simulink model "comparando_simulacoes_rate_diferente_entre_sensor_e_controlador"  (R2012b)
settings: Solver=ode3  StartTime=0.0  StopTime=1  FixedStep=1e-5  RelTol=1e-6
undefined symbols (not defined in the file): J, Kd, Ke, Kt, L, P, R
libraries: simulink x86
(part 2 of 3)

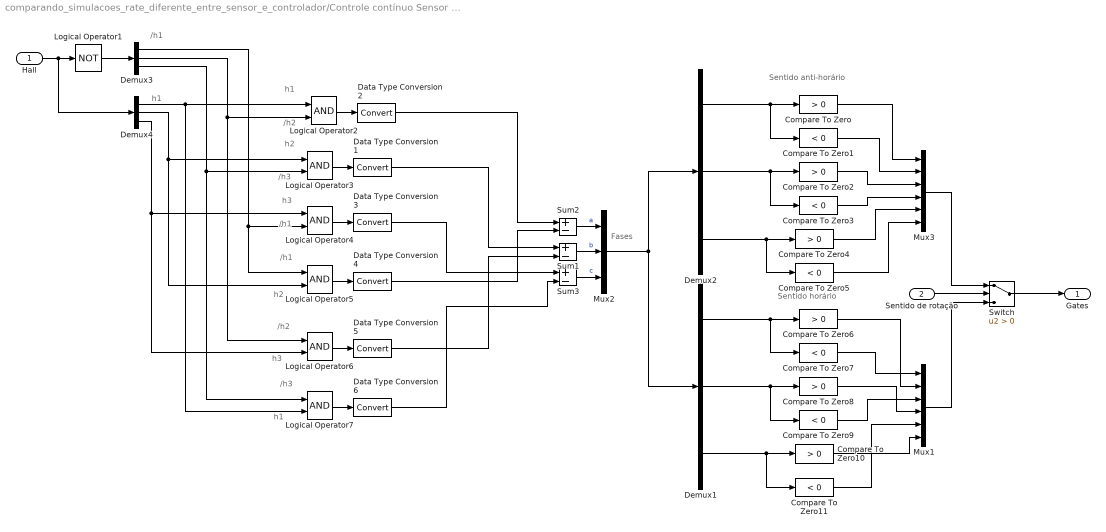
== system comparando_simulacoes_rate_diferente_entre_sensor_e_controlador/Controle contínuo Sensor instantâneo/Decoder ==
  note: Fases
  note: Sentido horário
  note: Sentido anti-horário
  note: h1
  note: /h3
  note: h3
  note: /h2
  note: h2
  note: /h1
  note: /h1
  note: h3
  note: /h3
  note: h2
  note: /h2
  note: h1
  note: h1
  note: /h1
  "Hall " : Inport
  Sentido de rotação : Inport  Port=2
  Compare To Zero{,2,4,6,8,10} (6 alike) : simulink/Logic and Bit Operations/Compare To Zero  relop=>  OutDataTypeStr=boolean  ZeroCross=off
  Compare To Zero{1,3,5,7,9,11} (6 alike) : simulink/Logic and Bit Operations/Compare To Zero  relop=<  OutDataTypeStr=boolean  ZeroCross=off
  Data Type Conversion{1..6} (6 alike) : DataTypeConversion
  Demux{1..4} (4 alike) : Demux  Outputs=3
  Logical Operator1 : Logic  Operator=NOT  AllPortsSameDT=off  OutDataTypeStr=boolean
  Logical Operator{2..7} (6 alike) : Logic  AllPortsSameDT=off  OutDataTypeStr=boolean
  Mux1 : Mux  Inputs=6
  Mux2 : Mux  Inputs=3
  Mux3 : Mux  Inputs=6
  Sum1 : Sum  Inputs=+-  OutDataTypeStr=double
  Sum2 : Sum  Inputs=+-  OutDataTypeStr=double
  Sum3 : Sum  Inputs=+-  OutDataTypeStr=double
  Switch : Switch  Criteria=u2 > Threshold
  Gates : Outport
  wires:
  Mux2/1 -> Demux1/1, Demux2/1
  Data Type Conversion6/1 -> Sum3/2
  Data Type Conversion3/1 -> Sum3/1
  Data Type Conversion5/1 -> Sum1/2
  Data Type Conversion1/1 -> Sum1/1
  Data Type Conversion4/1 -> Sum2/2
  Data Type Conversion2/1 -> Sum2/1
  Logical Operator7/1 -> Data Type Conversion6/1
  Logical Operator6/1 -> Data Type Conversion5/1
  Logical Operator5/1 -> Data Type Conversion4/1
  Logical Operator4/1 -> Data Type Conversion3/1
  Logical Operator3/1 -> Data Type Conversion1/1
  Sum3/1 -> Mux2/3  "c"
  Sum1/1 -> Mux2/2  "b"
  Sum2/1 -> Mux2/1  "a"
  Logical Operator2/1 -> Data Type Conversion2/1
  Demux3/1 -> Logical Operator5/1, Logical Operator4/2
  Demux3/2 -> Logical Operator6/1, Logical Operator2/2
  Demux3/3 -> Logical Operator7/1, Logical Operator3/2
  Demux4/1 -> Logical Operator7/2, Logical Operator2/1
  Demux4/2 -> Logical Operator5/2, Logical Operator3/1
  Demux4/3 -> Logical Operator6/2, Logical Operator4/1
  Logical Operator1/1 -> Demux3/1
  "Hall "/1 -> Demux4/1, Logical Operator1/1
  Compare To Zero10/1 -> Mux1/6
  Compare To Zero11/1 -> Mux1/5
  Compare To Zero8/1 -> Mux1/4
  Compare To Zero9/1 -> Mux1/3
  Compare To Zero6/1 -> Mux1/2
  Compare To Zero7/1 -> Mux1/1
  Switch/1 -> Gates/1
  Mux1/1 -> Switch/3
  Sentido de rotação/1 -> Switch/2
  Mux3/1 -> Switch/1
  Demux1/3 -> Compare To Zero11/1, Compare To Zero10/1
  Demux1/2 -> Compare To Zero9/1, Compare To Zero8/1
  Demux1/1 -> Compare To Zero7/1, Compare To Zero6/1
  Compare To Zero5/1 -> Mux3/6
  Compare To Zero4/1 -> Mux3/5
  Compare To Zero3/1 -> Mux3/4
  Compare To Zero2/1 -> Mux3/3
  Compare To Zero1/1 -> Mux3/2
  Compare To Zero/1 -> Mux3/1
  Demux2/3 -> Compare To Zero5/1, Compare To Zero4/1
  Demux2/2 -> Compare To Zero3/1, Compare To Zero2/1
  Demux2/1 -> Compare To Zero1/1, Compare To Zero/1

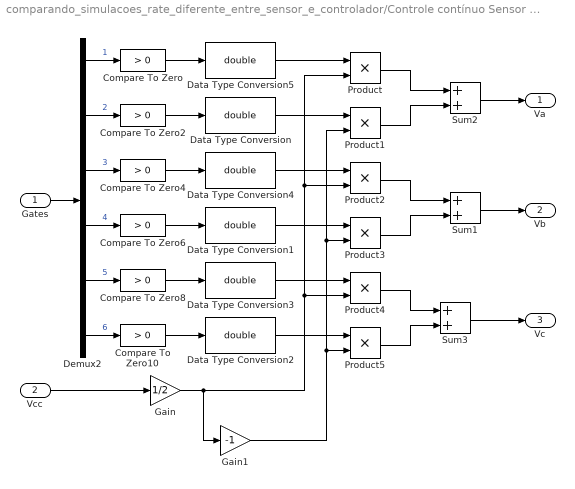
== system comparando_simulacoes_rate_diferente_entre_sensor_e_controlador/Controle contínuo Sensor instantâneo/Inversor ==
  Gates : Inport
  Vcc : Inport  Port=2
  Compare To Zero : simulink/Logic and Bit Operations/Compare To Zero  relop=>  OutDataTypeStr=uint8  ZeroCross=off
  Compare To Zero{2,6,8,10} (4 alike) : simulink/Logic and Bit Operations/Compare To Zero  relop=>  OutDataTypeStr=boolean  ZeroCross=off
  Compare To Zero4 : simulink/Logic and Bit Operations/Compare To Zero  relop=>  OutDataTypeStr=uint8  ZeroCross=off
  Data Type Conversion{,1..5} (6 alike) : DataTypeConversion  OutDataTypeStr=double
  Demux2 : Demux  Outputs=6
  Gain : Gain  Gain=1/2
  Gain1 : Gain  Gain=-1
  Product{,1..5} (6 alike) : Product  RndMeth=Zero
  Sum1 : Sum  SaturateOnIntegerOverflow=on
  Sum2 : Sum  SaturateOnIntegerOverflow=on
  Sum3 : Sum  SaturateOnIntegerOverflow=on
  Va : Outport
  Vb : Outport  Port=2
  Vc : Outport  Port=3
  wires:
  Vcc/1 -> Gain/1
  Sum1/1 -> Vb/1
  Sum3/1 -> Vc/1
  Sum2/1 -> Va/1
  Gates/1 -> Demux2/1
  Demux2/1 -> Compare To Zero/1  "1"
  Demux2/2 -> Compare To Zero2/1  "2"
  Demux2/3 -> Compare To Zero4/1  "3"
  Demux2/4 -> Compare To Zero6/1  "4"
  Demux2/5 -> Compare To Zero8/1  "5"
  Demux2/6 -> Compare To Zero10/1  "6"
  Compare To Zero/1 -> Data Type Conversion5/1
  Compare To Zero2/1 -> Data Type Conversion/1
  Compare To Zero4/1 -> Data Type Conversion4/1
  Compare To Zero6/1 -> Data Type Conversion1/1
  Compare To Zero8/1 -> Data Type Conversion3/1
  Compare To Zero10/1 -> Data Type Conversion2/1
  Product/1 -> Sum2/1
  Product1/1 -> Sum2/2
  Product2/1 -> Sum1/1
  Product3/1 -> Sum1/2
  Product4/1 -> Sum3/1
  Product5/1 -> Sum3/2
  Data Type Conversion2/1 -> Product5/1
  Data Type Conversion3/1 -> Product4/1
  Data Type Conversion1/1 -> Product3/1
  Data Type Conversion4/1 -> Product2/1
  Data Type Conversion/1 -> Product1/1
  Data Type Conversion5/1 -> Product/1
  Gain1/1 -> Product5/2, Product3/2, Product1/2
  Gain/1 -> Gain1/1, Product4/2, Product2/2, Product/2

== system comparando_simulacoes_rate_diferente_entre_sensor_e_controlador/Controle contínuo Sensor instantâneo/Sensores Hall ==
  teta_e : Inport
  Constant10 : Constant  Value=240
  Constant11 : Constant  Value=360
  Constant12 : Constant  Value=180
  Constant6 : Constant  Value=0
  Constant7 : Constant  Value=120
  Constant8 : Constant  Value=300
  Constant9 : Constant  Value=60
  Data Type Conversion3 : DataTypeConversion  SaturateOnIntegerOverflow=on  RndMeth=Zero
  Data Type Conversion4 : DataTypeConversion  SaturateOnIntegerOverflow=on  RndMeth=Zero
  Data Type Conversion5 : DataTypeConversion  SaturateOnIntegerOverflow=on  RndMeth=Zero
  Gain1 : Gain  Gain=180/pi
  Logical Operator3 : Logic  AllPortsSameDT=off  OutDataTypeStr=boolean
  Logical Operator4 : Logic  Operator=OR  AllPortsSameDT=off  OutDataTypeStr=boolean
  Logical Operator5 : Logic  AllPortsSameDT=off  OutDataTypeStr=boolean
  Math Function1 : Math  Operator=mod  SaturateOnIntegerOverflow=on
  Mux1 : Mux  Inputs=3
  Relational Operator{7,9..10,12} (4 alike) : RelationalOperator  InputSameDT=on
  Relational Operator11 : RelationalOperator  Operator=<=  InputSameDT=on
  Relational Operator8 : RelationalOperator  Operator=<=  InputSameDT=on
  Hall : Outport
  wires:
  teta_e/1 -> Gain1/1
  Constant6/1 -> Relational Operator7/2
  Constant7/1 -> Relational Operator8/2
  Constant8/1 -> Relational Operator9/2
  Relational Operator9/1 -> Logical Operator4/2
  Logical Operator3/1 -> Logical Operator4/1
  Relational Operator7/1 -> Logical Operator3/1
  Relational Operator8/1 -> Logical Operator3/2
  Relational Operator10/1 -> Logical Operator5/1
  Relational Operator11/1 -> Logical Operator5/2
  Constant9/1 -> Relational Operator10/2
  Constant10/1 -> Relational Operator11/2
  Constant12/1 -> Relational Operator12/2
  Mux1/1 -> Hall/1
  Data Type Conversion3/1 -> Mux1/1
  Data Type Conversion4/1 -> Mux1/2
  Data Type Conversion5/1 -> Mux1/3
  Logical Operator4/1 -> Data Type Conversion3/1
  Logical Operator5/1 -> Data Type Conversion4/1
  Relational Operator12/1 -> Data Type Conversion5/1
  Gain1/1 -> Math Function1/1
  Constant11/1 -> Math Function1/2
  Math Function1/1 -> Relational Operator8/1, Relational Operator9/1, Relational Operator10/1, Relational Operator11/1, Relational Operator12/1, Relational Operator7/1

== system comparando_simulacoes_rate_diferente_entre_sensor_e_controlador/Controlador contínuo Sensor discreto M (Ts = 0.01)/BLDC1/Cálculo Torque fase "a" ==
  i_a : Inport
  Theta_e : Inport  Port=2
  Constant1 : Constant  Value=360
  Gain : Gain  Gain=Kt/2
  Gain1 : Gain  Gain=180/pi
  Math Function1 : Math  Operator=mod  SaturateOnIntegerOverflow=on
  Product : Product  RndMeth=Zero
  fa1 : Lookup  InputValues=[0 30 60 90 120 150 180 210 240 270 300 330 360]  Table=[ 1 1 1 0 -1 -1 -1 -1 -1 0 1 1 1]
  T_a : Outport
  wires:
  i_a/1 -> Gain/1
  Gain/1 -> Product/2
  Math Function1/1 -> fa1/1
  Theta_e/1 -> Gain1/1
  fa1/1 -> Product/1
  Product/1 -> T_a/1
  Gain1/1 -> Math Function1/1
  Constant1/1 -> Math Function1/2

== system comparando_simulacoes_rate_diferente_entre_sensor_e_controlador/Controlador contínuo Sensor discreto M (Ts = 0.01)/BLDC1/Cálculo Torque fase "b" ==
  i_b : Inport
  Theta_e : Inport  Port=2
  Constant1 : Constant  Value=360
  Gain : Gain  Gain=Kt/2
  Gain1 : Gain  Gain=180/pi
  Math Function1 : Math  Operator=mod  SaturateOnIntegerOverflow=on
  Product : Product  RndMeth=Zero
  fb2 : Lookup  InputValues=[0 30 60 90 120 150 180 210 240 270 300 330 360]  Table=[-1 0 1 1 1 1 1 0 -1 -1 -1 -1 -1]
  T_b : Outport
  wires:
  Product/1 -> T_b/1
  fb2/1 -> Product/1
  Theta_e/1 -> Gain1/1
  Math Function1/1 -> fb2/1
  Gain/1 -> Product/2
  i_b/1 -> Gain/1
  Gain1/1 -> Math Function1/1
  Constant1/1 -> Math Function1/2

== system comparando_simulacoes_rate_diferente_entre_sensor_e_controlador/Controlador contínuo Sensor discreto M (Ts = 0.01)/BLDC1/Cálculo Torque fase "c" ==
  i_c : Inport
  Theta_e : Inport  Port=2
  Constant1 : Constant  Value=360
  Gain : Gain  Gain=Kt/2
  Gain1 : Gain  Gain=180/pi
  Math Function1 : Math  Operator=mod  SaturateOnIntegerOverflow=on
  Product : Product  RndMeth=Zero
  fc1 : Lookup  InputValues=[0 30 60 90 120 150 180 210 240 270 300 330 360]  Table=[-1 -1 -1 -1 -1 0 1 1 1 1 1 0 -1]
  T_c : Outport
  wires:
  i_c/1 -> Gain/1
  Gain/1 -> Product/2
  Math Function1/1 -> fc1/1
  Theta_e/1 -> Gain1/1
  fc1/1 -> Product/1
  Product/1 -> T_c/1
  Gain1/1 -> Math Function1/1
  Constant1/1 -> Math Function1/2

== system comparando_simulacoes_rate_diferente_entre_sensor_e_controlador/Controlador contínuo Sensor discreto M (Ts = 0.01)/BLDC1/Cálculo das FCEMs ==
  Theta_e : Inport
  w_m : Inport  Port=2
  Constant1 : Constant  Value=360
  Constant2 : Constant  Value=360
  Constant3 : Constant  Value=360
  Gain1 : Gain  Gain=180/pi
  Gain2 : Gain  Gain=Ke/2
  Gain3 : Gain  Gain=Ke/2
  Gain4 : Gain  Gain=Ke/2
  Gain5 : Gain  Gain=180/pi
  Gain6 : Gain  Gain=180/pi
  Math Function1 : Math  Operator=mod  SaturateOnIntegerOverflow=on
  Math Function2 : Math  Operator=mod  SaturateOnIntegerOverflow=on
  Math Function3 : Math  Operator=mod  SaturateOnIntegerOverflow=on
  Product : Product  RndMeth=Zero
  Product1 : Product  RndMeth=Zero
  Product2 : Product  RndMeth=Zero
  fa1 : Lookup  InputValues=[0 30 60 90 120 150 180 210 240 270 300 330 360]  Table=[ 1 1 1 0 -1 -1 -1 -1 -1 0 1 1 1]
  fb2 : Lookup  InputValues=[0 30 60 90 120 150 180 210 240 270 300 330 360]  Table=[-1 0 1 1 1 1 1 0 -1 -1 -1 -1 -1]
  fc1 : Lookup  InputValues=[0 30 60 90 120 150 180 210 240 270 300 330 360]  Table=[-1 -1 -1 -1 -1 0 1 1 1 1 1 0 -1]
  e_a : Outport
  e_b : Outport  Port=2
  e_c : Outport  Port=3
  wires:
  fc1/1 -> Gain4/1
  Math Function3/1 -> fc1/1
  fb2/1 -> Gain3/1
  Math Function2/1 -> fb2/1
  fa1/1 -> Gain2/1
  Math Function1/1 -> fa1/1
  Gain6/1 -> Math Function3/1
  Gain5/1 -> Math Function2/1
  Gain1/1 -> Math Function1/1
  Gain4/1 -> Product2/2
  Gain3/1 -> Product1/2
  w_m/1 -> Product2/1, Product1/1, Product/1
  Gain2/1 -> Product/2
  Product2/1 -> e_c/1
  Theta_e/1 -> Gain6/1, Gain1/1, Gain5/1
  Product1/1 -> e_b/1
  Product/1 -> e_a/1
  Constant1/1 -> Math Function1/2
  Constant2/1 -> Math Function2/2
  Constant3/1 -> Math Function3/2

== system comparando_simulacoes_rate_diferente_entre_sensor_e_controlador/Controlador contínuo Sensor discreto M (Ts = 0.01)/BLDC1/Dinâmica fase "a" ==
  note: Gain
  Va : Inport
  e_a : Inport  Port=2
  " " : Gain  Gain=1/L
  Gain : Gain  Gain=R
  Integrator : Integrator
  Sum : Sum  Inputs=+--
  i_a : Outport
  wires:
  Integrator/1 -> i_a/1, Gain/1
  Va/1 -> Sum/1
  Sum/1 -> " "/1
  " "/1 -> Integrator/1
  Gain/1 -> Sum/3
  e_a/1 -> Sum/2

== system comparando_simulacoes_rate_diferente_entre_sensor_e_controlador/Controlador contínuo Sensor discreto M (Ts = 0.01)/BLDC1/Dinâmica fase "b" ==
  note: Gain
  Vb : Inport
  e_b : Inport  Port=2
  " " : Gain  Gain=1/L
  Gain : Gain  Gain=R
  Integrator : Integrator
  Sum : Sum  Inputs=+--
  i_b : Outport
  wires:
  e_b/1 -> Sum/2
  Gain/1 -> Sum/3
  " "/1 -> Integrator/1
  Sum/1 -> " "/1
  Vb/1 -> Sum/1
  Integrator/1 -> Gain/1, i_b/1

== system comparando_simulacoes_rate_diferente_entre_sensor_e_controlador/Controlador contínuo Sensor discreto M (Ts = 0.01)/BLDC1/Dinâmica fase "c" ==
  note: Gain
  Vc : Inport
  e_c : Inport  Port=2
  " " : Gain  Gain=1/L
  Gain : Gain  Gain=R
  Integrator : Integrator
  Sum : Sum  Inputs=+--
  i_c : Outport
  wires:
  Integrator/1 -> i_c/1, Gain/1
  Vc/1 -> Sum/1
  Sum/1 -> " "/1
  " "/1 -> Integrator/1
  Gain/1 -> Sum/3
  e_c/1 -> Sum/2

== system comparando_simulacoes_rate_diferente_entre_sensor_e_controlador/Controlador contínuo Sensor discreto M (Ts = 0.01)/BLDC1/Dinâmica mecânica  ==
  Te : Inport
  Tl : Inport  Port=2
  Gain : Gain  Gain=1/J
  Gain1 : Gain  Gain=Kd
  Integrator : Integrator
  Integrator1 : Integrator
  Sum1 : Sum  Inputs=+--
  Theta_m : Outport
  w_m : Outport  Port=2
  wires:
  Sum1/1 -> Gain/1
  Gain/1 -> Integrator/1
  Integrator/1 -> w_m/1, Integrator1/1, Gain1/1
  Te/1 -> Sum1/1
  Gain1/1 -> Sum1/3
  Tl/1 -> Sum1/2
  Integrator1/1 -> Theta_m/1

== system comparando_simulacoes_rate_diferente_entre_sensor_e_controlador/Controlador contínuo Sensor discreto M (Ts = 0.01)/Encoder/Determinar direçao ==
  note: Dependendo dos valores passados e dos valores atuais
      | dos pulsos de cada sensor óptico, determina o sentido
      | de rotaçao.
  note: 00
      | 01
      | 10
      | 11
  note: 00 01 10 11
  note: 0	-	+	0
      | +	0	0	-
      | -	0	0	+
      | 0	+	-	0
  note: Implementa a seguinte tabela verdade:
  note: AB
  note: A'B'
  note: A,B = Valores atuais dos sinais A e B
      | A'B' = Valores passados do sinais A e B
  A : Inport
  B : Inport  Port=2
  Bus Creator1 : BusCreator
  Combinatorial  Logic : CombinatorialLogic  TruthTable=[ 0 0 ; 0 1 ; 1 0 ; 0 0 ; 1 0 ; 0 0 ; 0 0 ; 0 1 ; 0 1 ; 0 0 ; 0 0 ; 1 0 ; 0 0 ; 1 0 ; 0 1 ; 0 0]
  Demux : Demux  Outputs=2
  Memory : Memory
  Memory1 : Memory
  POS : Outport
  NEG : Outport  Port=2
  wires:
  B/1 -> Bus Creator1/4, Memory1/1
  Memory1/1 -> Bus Creator1/2
  Bus Creator1/1 -> Combinatorial  Logic/1
  Memory/1 -> Bus Creator1/1
  Combinatorial  Logic/1 -> Demux/1
  Demux/2 -> NEG/1
  A/1 -> Bus Creator1/3, Memory/1
  Demux/1 -> POS/1

== system comparando_simulacoes_rate_diferente_entre_sensor_e_controlador/Controlador contínuo Sensor discreto M (Ts = 0.01)/Encoder/Método M ==
  Posição : Inport
  Add : Sum  Inputs=+-|
  Detect Increase : simulink/Logic and Bit Operations/Detect Increase  vinit=0.0  InputProcessing=Inherited  OutDataTypeStr=boolean
  Gain : Gain  Gain=1/Ts
  Memory1 : Memory
  Pulse Generator : DiscretePulseGenerator  PulseType=Time based  Period=Ts  PulseWidth=50
  Switch : Switch
  Switch1 : Switch
  pos' : Memory
  Velocidade : Outport
  wires:
  Detect Increase/1 -> Switch1/2, Switch/2
  Gain/1 -> Switch/1
  Posição/1 -> Add/1, Switch1/1
  Memory1/1 -> Switch/3, Velocidade/1
  Switch/1 -> Memory1/1
  Switch1/1 -> pos'/1
  Add/1 -> Gain/1
  Pulse Generator/1 -> Detect Increase/1
  pos'/1 -> Switch1/3, Add/2

== system comparando_simulacoes_rate_diferente_entre_sensor_e_controlador/Controlador contínuo Sensor discreto M (Ts = 0.01)/Encoder/Método T ==
  A : Inport
  B : Inport  Port=2
  Clock : Clock
  Compare To Constant : simulink/Logic and Bit Operations/Compare To Constant  relop===  const=m  OutDataTypeStr=boolean
  Constant : Constant  Value=m
  Contador : Subsystem
  Detect Change : simulink/Logic and Bit Operations/Detect Change  vinit=0  InputProcessing=Inherited  OutDataTypeStr=boolean
  Detect Change1 : simulink/Logic and Bit Operations/Detect Change  vinit=0  InputProcessing=Inherited  OutDataTypeStr=boolean
  Divide : Product  Inputs=*/
  Gain : Gain  Gain=360/(4*Nr)
  Logical Operator : Logic  Operator=OR  AllPortsSameDT=off  OutDataTypeStr=boolean
  Memória controlavel : Subsystem
  Memória controlavel1 : Subsystem
  Sum : Sum  Inputs=|+-
  Velocidade : Outport
  wires:
  Memória controlavel1/1(Out) -> Velocidade/1
  Compare To Constant/1 -> Memória controlavel/2(ctrl), Contador/2(reset), Memória controlavel1/2(ctrl)
  Clock/1 -> Memória controlavel/1(In), Sum/1
  Gain/1 -> Divide/1
  Sum/1 -> Divide/2
  Memória controlavel/1(Out) -> Sum/2
  Divide/1 -> Memória controlavel1/1(In)
  Constant/1 -> Gain/1
  Contador/1(Count) -> Compare To Constant/1
  Logical Operator/1 -> Contador/1(In)
  Detect Change1/1 -> Logical Operator/2
  Detect Change/1 -> Logical Operator/1
  B/1 -> Detect Change1/1
  A/1 -> Detect Change/1

== system comparando_simulacoes_rate_diferente_entre_sensor_e_controlador/Controlador contínuo Sensor discreto M (Ts = 0.01)/Encoder/Sensor Óptico ==
  note: Saída do sensor óptico é:
      | 1, se	0 < mod(T,Tp) < \frac{Tp}{2}
      |  0, se      Tp/2 < mod(T,Tp) < Tp
  Theta : Inport
  Constant : Constant  Value=0
  Constant1 : Constant  Value=Nr
  Constant2 : Constant  Value=360
  Divide : Product  Inputs=*/
  Gain : Gain  Gain=1/2
  Logical Operator : Logic  AllPortsSameDT=off  OutDataTypeStr=boolean
  Math Function : Math  Operator=mod  SaturateOnIntegerOverflow=on
  Relational Operator : RelationalOperator  Operator=>  OutDataTypeStr=boolean
  Relational Operator1 : RelationalOperator  Operator=<  OutDataTypeStr=boolean
  Sinal_Pulso : Outport
  wires:
  Constant1/1 -> Divide/2
  Constant2/1 -> Divide/1
  Logical Operator/1 -> Sinal_Pulso/1
  Gain/1 -> Relational Operator1/2
  Divide/1 -> Gain/1, Math Function/2  "Theta_p"
  Constant/1 -> Relational Operator/2
  Relational Operator1/1 -> Logical Operator/2
  Relational Operator/1 -> Logical Operator/1
  Theta/1 -> Math Function/1
  Math Function/1 -> Relational Operator/1, Relational Operator1/1

== system comparando_simulacoes_rate_diferente_entre_sensor_e_controlador/Controlador contínuo Sensor discreto M (Ts = 0.01)/Encoder/Sensor Óptico1 ==
  note: Saída do sensor óptico é:
      | 1, se	0 < mod(T-Tp/4,Tp) < Tp/2
      |  0, se     Tp/2 < mod(T-Tp/4,Tp) < Tp
  Theta : Inport
  Add : Sum  Inputs=+-
  Constant : Constant  Value=0
  Constant1 : Constant  Value=Nr
  Constant2 : Constant  Value=360
  Divide : Product  Inputs=*/
  Gain : Gain  Gain=1/2
  Gain1 : Gain  Gain=1/4
  Logical Operator : Logic  AllPortsSameDT=off  OutDataTypeStr=boolean
  Math Function : Math  Operator=mod  SaturateOnIntegerOverflow=on
  Relational Operator : RelationalOperator  Operator=>  OutDataTypeStr=boolean
  Relational Operator1 : RelationalOperator  Operator=<  OutDataTypeStr=boolean
  Sinal_Pulso : Outport
  wires:
  Gain1/1 -> Add/2
  Theta/1 -> Add/1
  Add/1 -> Math Function/1
  Math Function/1 -> Relational Operator1/1, Relational Operator/1
  Relational Operator/1 -> Logical Operator/1
  Relational Operator1/1 -> Logical Operator/2
  Constant/1 -> Relational Operator/2
  Divide/1 -> Math Function/2, Gain/1, Gain1/1  "Theta_p"
  Gain/1 -> Relational Operator1/2
  Logical Operator/1 -> Sinal_Pulso/1
  Constant2/1 -> Divide/1
  Constant1/1 -> Divide/2

== system comparando_simulacoes_rate_diferente_entre_sensor_e_controlador/Controlador contínuo Sensor discreto M (Ts = 0.01)/Encoder/Subsystem ==
  note: Dependendo do sentido da rotaçao, incrementa ou decrementa o contador
  POS : Inport
  NEG : Inport  Port=2
  Constant : Constant  Value=4*Nr
  Conversion : DataTypeConversion  OutDataTypeStr=int32
  Conversion1 : DataTypeConversion  OutDataTypeStr=int32
  Math Function : Math  Operator=mod  SaturateOnIntegerOverflow=on
  Memory : Memory
  Sum : Sum  Inputs=+-+
  Out : Outport
  wires:
  NEG/1 -> Conversion1/1
  Conversion1/1 -> Sum/2
  Conversion/1 -> Sum/1
  POS/1 -> Conversion/1
  Math Function/1 -> Memory/1
  Memory/1 -> Sum/3, Out/1
  Sum/1 -> Math Function/1

== system comparando_simulacoes_rate_diferente_entre_sensor_e_controlador/Controlador discreto (Ts = 0.001) Sensor discreto M (Ts = 0.01)/BLDC1/Cálculo Torque fase "a" ==
  i_a : Inport
  Theta_e : Inport  Port=2
  Constant1 : Constant  Value=360
  Gain : Gain  Gain=Kt/2
  Gain1 : Gain  Gain=180/pi
  Math Function1 : Math  Operator=mod  SaturateOnIntegerOverflow=on
  Product : Product  RndMeth=Zero
  fa1 : Lookup  InputValues=[0 30 60 90 120 150 180 210 240 270 300 330 360]  Table=[ 1 1 1 0 -1 -1 -1 -1 -1 0 1 1 1]
  T_a : Outport
  wires:
  Constant1/1 -> Math Function1/2
  Gain1/1 -> Math Function1/1
  Product/1 -> T_a/1
  fa1/1 -> Product/1
  Theta_e/1 -> Gain1/1
  Math Function1/1 -> fa1/1
  Gain/1 -> Product/2
  i_a/1 -> Gain/1

== system comparando_simulacoes_rate_diferente_entre_sensor_e_controlador/Controlador discreto (Ts = 0.001) Sensor discreto M (Ts = 0.01)/BLDC1/Cálculo Torque fase "b" ==
  i_b : Inport
  Theta_e : Inport  Port=2
  Constant1 : Constant  Value=360
  Gain : Gain  Gain=Kt/2
  Gain1 : Gain  Gain=180/pi
  Math Function1 : Math  Operator=mod  SaturateOnIntegerOverflow=on
  Product : Product  RndMeth=Zero
  fb2 : Lookup  InputValues=[0 30 60 90 120 150 180 210 240 270 300 330 360]  Table=[-1 0 1 1 1 1 1 0 -1 -1 -1 -1 -1]
  T_b : Outport
  wires:
  Constant1/1 -> Math Function1/2
  Gain1/1 -> Math Function1/1
  i_b/1 -> Gain/1
  Gain/1 -> Product/2
  Math Function1/1 -> fb2/1
  Theta_e/1 -> Gain1/1
  fb2/1 -> Product/1
  Product/1 -> T_b/1

== system comparando_simulacoes_rate_diferente_entre_sensor_e_controlador/Controlador discreto (Ts = 0.001) Sensor discreto M (Ts = 0.01)/BLDC1/Cálculo Torque fase "c" ==
  i_c : Inport
  Theta_e : Inport  Port=2
  Constant1 : Constant  Value=360
  Gain : Gain  Gain=Kt/2
  Gain1 : Gain  Gain=180/pi
  Math Function1 : Math  Operator=mod  SaturateOnIntegerOverflow=on
  Product : Product  RndMeth=Zero
  fc1 : Lookup  InputValues=[0 30 60 90 120 150 180 210 240 270 300 330 360]  Table=[-1 -1 -1 -1 -1 0 1 1 1 1 1 0 -1]
  T_c : Outport
  wires:
  Constant1/1 -> Math Function1/2
  Gain1/1 -> Math Function1/1
  Product/1 -> T_c/1
  fc1/1 -> Product/1
  Theta_e/1 -> Gain1/1
  Math Function1/1 -> fc1/1
  Gain/1 -> Product/2
  i_c/1 -> Gain/1

== system comparando_simulacoes_rate_diferente_entre_sensor_e_controlador/Controlador discreto (Ts = 0.001) Sensor discreto M (Ts = 0.01)/BLDC1/Cálculo das FCEMs ==
  Theta_e : Inport
  w_m : Inport  Port=2
  Constant1 : Constant  Value=360
  Constant2 : Constant  Value=360
  Constant3 : Constant  Value=360
  Gain1 : Gain  Gain=180/pi
  Gain2 : Gain  Gain=Ke/2
  Gain3 : Gain  Gain=Ke/2
  Gain4 : Gain  Gain=Ke/2
  Gain5 : Gain  Gain=180/pi
  Gain6 : Gain  Gain=180/pi
  Math Function1 : Math  Operator=mod  SaturateOnIntegerOverflow=on
  Math Function2 : Math  Operator=mod  SaturateOnIntegerOverflow=on
  Math Function3 : Math  Operator=mod  SaturateOnIntegerOverflow=on
  Product : Product  RndMeth=Zero
  Product1 : Product  RndMeth=Zero
  Product2 : Product  RndMeth=Zero
  fa1 : Lookup  InputValues=[0 30 60 90 120 150 180 210 240 270 300 330 360]  Table=[ 1 1 1 0 -1 -1 -1 -1 -1 0 1 1 1]
  fb2 : Lookup  InputValues=[0 30 60 90 120 150 180 210 240 270 300 330 360]  Table=[-1 0 1 1 1 1 1 0 -1 -1 -1 -1 -1]
  fc1 : Lookup  InputValues=[0 30 60 90 120 150 180 210 240 270 300 330 360]  Table=[-1 -1 -1 -1 -1 0 1 1 1 1 1 0 -1]
  e_a : Outport
  e_b : Outport  Port=2
  e_c : Outport  Port=3
  wires:
  Constant3/1 -> Math Function3/2
  Constant2/1 -> Math Function2/2
  Constant1/1 -> Math Function1/2
  Product/1 -> e_a/1
  Product1/1 -> e_b/1
  Theta_e/1 -> Gain5/1, Gain1/1, Gain6/1
  Product2/1 -> e_c/1
  Gain2/1 -> Product/2
  w_m/1 -> Product/1, Product1/1, Product2/1
  Gain3/1 -> Product1/2
  Gain4/1 -> Product2/2
  Gain1/1 -> Math Function1/1
  Gain5/1 -> Math Function2/1
  Gain6/1 -> Math Function3/1
  Math Function1/1 -> fa1/1
  fa1/1 -> Gain2/1
  Math Function2/1 -> fb2/1
  fb2/1 -> Gain3/1
  Math Function3/1 -> fc1/1
  fc1/1 -> Gain4/1

== system comparando_simulacoes_rate_diferente_entre_sensor_e_controlador/Controlador discreto (Ts = 0.001) Sensor discreto M (Ts = 0.01)/BLDC1/Dinâmica fase "a" ==
  note: Gain
  Va : Inport
  e_a : Inport  Port=2
  " " : Gain  Gain=1/L
  Gain : Gain  Gain=R
  Integrator : Integrator
  Sum : Sum  Inputs=+--
  i_a : Outport
  wires:
  e_a/1 -> Sum/2
  Gain/1 -> Sum/3
  " "/1 -> Integrator/1
  Sum/1 -> " "/1
  Va/1 -> Sum/1
  Integrator/1 -> Gain/1, i_a/1

== system comparando_simulacoes_rate_diferente_entre_sensor_e_controlador/Controlador discreto (Ts = 0.001) Sensor discreto M (Ts = 0.01)/BLDC1/Dinâmica fase "b" ==
  note: Gain
  Vb : Inport
  e_b : Inport  Port=2
  " " : Gain  Gain=1/L
  Gain : Gain  Gain=R
  Integrator : Integrator
  Sum : Sum  Inputs=+--
  i_b : Outport
  wires:
  Integrator/1 -> i_b/1, Gain/1
  Vb/1 -> Sum/1
  Sum/1 -> " "/1
  " "/1 -> Integrator/1
  Gain/1 -> Sum/3
  e_b/1 -> Sum/2

== system comparando_simulacoes_rate_diferente_entre_sensor_e_controlador/Controlador discreto (Ts = 0.001) Sensor discreto M (Ts = 0.01)/BLDC1/Dinâmica fase "c" ==
  note: Gain
  Vc : Inport
  e_c : Inport  Port=2
  " " : Gain  Gain=1/L
  Gain : Gain  Gain=R
  Integrator : Integrator
  Sum : Sum  Inputs=+--
  i_c : Outport
  wires:
  e_c/1 -> Sum/2
  Gain/1 -> Sum/3
  " "/1 -> Integrator/1
  Sum/1 -> " "/1
  Vc/1 -> Sum/1
  Integrator/1 -> Gain/1, i_c/1

== system comparando_simulacoes_rate_diferente_entre_sensor_e_controlador/Controlador discreto (Ts = 0.001) Sensor discreto M (Ts = 0.01)/BLDC1/Dinâmica mecânica  ==
  Te : Inport
  Tl : Inport  Port=2
  Gain : Gain  Gain=1/J
  Gain1 : Gain  Gain=Kd
  Integrator : Integrator
  Integrator1 : Integrator
  Sum1 : Sum  Inputs=+--
  Theta_m : Outport
  w_m : Outport  Port=2
  wires:
  Integrator1/1 -> Theta_m/1
  Tl/1 -> Sum1/2
  Gain1/1 -> Sum1/3
  Te/1 -> Sum1/1
  Integrator/1 -> Gain1/1, Integrator1/1, w_m/1
  Gain/1 -> Integrator/1
  Sum1/1 -> Gain/1

== system comparando_simulacoes_rate_diferente_entre_sensor_e_controlador/Controlador discreto (Ts = 0.001) Sensor discreto M (Ts = 0.01)/Encoder/Determinar direçao ==
  note: A,B = Valores atuais dos sinais A e B
      | A'B' = Valores passados do sinais A e B
  note: A'B'
  note: AB
  note: Implementa a seguinte tabela verdade:
  note: 0	-	+	0
      | +	0	0	-
      | -	0	0	+
      | 0	+	-	0
  note: 00 01 10 11
  note: 00
      | 01
      | 10
      | 11
  note: Dependendo dos valores passados e dos valores atuais
      | dos pulsos de cada sensor óptico, determina o sentido
      | de rotaçao.
  A : Inport
  B : Inport  Port=2
  Bus Creator1 : BusCreator
  Combinatorial  Logic : CombinatorialLogic  TruthTable=[ 0 0 ; 0 1 ; 1 0 ; 0 0 ; 1 0 ; 0 0 ; 0 0 ; 0 1 ; 0 1 ; 0 0 ; 0 0 ; 1 0 ; 0 0 ; 1 0 ; 0 1 ; 0 0]
  Demux : Demux  Outputs=2
  Memory : Memory
  Memory1 : Memory
  POS : Outport
  NEG : Outport  Port=2
  wires:
  Demux/1 -> POS/1
  A/1 -> Memory/1, Bus Creator1/3
  Demux/2 -> NEG/1
  Combinatorial  Logic/1 -> Demux/1
  Memory/1 -> Bus Creator1/1
  Bus Creator1/1 -> Combinatorial  Logic/1
  Memory1/1 -> Bus Creator1/2
  B/1 -> Memory1/1, Bus Creator1/4

== system comparando_simulacoes_rate_diferente_entre_sensor_e_controlador/Controlador discreto (Ts = 0.001) Sensor discreto M (Ts = 0.01)/Encoder/Método M ==
  Posição : Inport
  Add : Sum  Inputs=+-|
  Detect Increase : simulink/Logic and Bit Operations/Detect Increase  vinit=0.0  InputProcessing=Inherited  OutDataTypeStr=boolean
  Gain : Gain  Gain=1/Ts
  Memory1 : Memory
  Pulse Generator : DiscretePulseGenerator  PulseType=Time based  Period=Ts  PulseWidth=50
  Switch : Switch
  Switch1 : Switch
  pos' : Memory
  Velocidade : Outport
  wires:
  pos'/1 -> Add/2, Switch1/3
  Pulse Generator/1 -> Detect Increase/1
  Add/1 -> Gain/1
  Switch1/1 -> pos'/1
  Switch/1 -> Memory1/1
  Memory1/1 -> Velocidade/1, Switch/3
  Posição/1 -> Switch1/1, Add/1
  Gain/1 -> Switch/1
  Detect Increase/1 -> Switch/2, Switch1/2

== system comparando_simulacoes_rate_diferente_entre_sensor_e_controlador/Controlador discreto (Ts = 0.001) Sensor discreto M (Ts = 0.01)/Encoder/Método T ==
  A : Inport
  B : Inport  Port=2
  Clock : Clock
  Compare To Constant : simulink/Logic and Bit Operations/Compare To Constant  relop===  const=m  OutDataTypeStr=boolean
  Constant : Constant  Value=m
  Contador : Subsystem
  Detect Change : simulink/Logic and Bit Operations/Detect Change  vinit=0  InputProcessing=Inherited  OutDataTypeStr=boolean
  Detect Change1 : simulink/Logic and Bit Operations/Detect Change  vinit=0  InputProcessing=Inherited  OutDataTypeStr=boolean
  Divide : Product  Inputs=*/
  Gain : Gain  Gain=360/(4*Nr)
  Logical Operator : Logic  Operator=OR  AllPortsSameDT=off  OutDataTypeStr=boolean
  Memória controlavel : Subsystem
  Memória controlavel1 : Subsystem
  Sum : Sum  Inputs=|+-
  Velocidade : Outport
  wires:
  A/1 -> Detect Change/1
  B/1 -> Detect Change1/1
  Detect Change/1 -> Logical Operator/1
  Detect Change1/1 -> Logical Operator/2
  Logical Operator/1 -> Contador/1(In)
  Contador/1(Count) -> Compare To Constant/1
  Constant/1 -> Gain/1
  Divide/1 -> Memória controlavel1/1(In)
  Memória controlavel/1(Out) -> Sum/2
  Sum/1 -> Divide/2
  Gain/1 -> Divide/1
  Clock/1 -> Sum/1, Memória controlavel/1(In)
  Compare To Constant/1 -> Memória controlavel1/2(ctrl), Contador/2(reset), Memória controlavel/2(ctrl)
  Memória controlavel1/1(Out) -> Velocidade/1

== system comparando_simulacoes_rate_diferente_entre_sensor_e_controlador/Controlador discreto (Ts = 0.001) Sensor discreto M (Ts = 0.01)/Encoder/Sensor Óptico ==
  note: Saída do sensor óptico é:
      | 1, se	0 < mod(T,Tp) < \frac{Tp}{2}
      |  0, se      Tp/2 < mod(T,Tp) < Tp
  Theta : Inport
  Constant : Constant  Value=0
  Constant1 : Constant  Value=Nr
  Constant2 : Constant  Value=360
  Divide : Product  Inputs=*/
  Gain : Gain  Gain=1/2
  Logical Operator : Logic  AllPortsSameDT=off  OutDataTypeStr=boolean
  Math Function : Math  Operator=mod  SaturateOnIntegerOverflow=on
  Relational Operator : RelationalOperator  Operator=>  OutDataTypeStr=boolean
  Relational Operator1 : RelationalOperator  Operator=<  OutDataTypeStr=boolean
  Sinal_Pulso : Outport
  wires:
  Math Function/1 -> Relational Operator1/1, Relational Operator/1
  Theta/1 -> Math Function/1
  Relational Operator/1 -> Logical Operator/1
  Relational Operator1/1 -> Logical Operator/2
  Constant/1 -> Relational Operator/2
  Divide/1 -> Math Function/2, Gain/1  "Theta_p"
  Gain/1 -> Relational Operator1/2
  Logical Operator/1 -> Sinal_Pulso/1
  Constant2/1 -> Divide/1
  Constant1/1 -> Divide/2

== system comparando_simulacoes_rate_diferente_entre_sensor_e_controlador/Controlador discreto (Ts = 0.001) Sensor discreto M (Ts = 0.01)/Encoder/Sensor Óptico1 ==
  note: Saída do sensor óptico é:
      | 1, se	0 < mod(T-Tp/4,Tp) < Tp/2
      |  0, se     Tp/2 < mod(T-Tp/4,Tp) < Tp
  Theta : Inport
  Add : Sum  Inputs=+-
  Constant : Constant  Value=0
  Constant1 : Constant  Value=Nr
  Constant2 : Constant  Value=360
  Divide : Product  Inputs=*/
  Gain : Gain  Gain=1/2
  Gain1 : Gain  Gain=1/4
  Logical Operator : Logic  AllPortsSameDT=off  OutDataTypeStr=boolean
  Math Function : Math  Operator=mod  SaturateOnIntegerOverflow=on
  Relational Operator : RelationalOperator  Operator=>  OutDataTypeStr=boolean
  Relational Operator1 : RelationalOperator  Operator=<  OutDataTypeStr=boolean
  Sinal_Pulso : Outport
  wires:
  Constant1/1 -> Divide/2
  Constant2/1 -> Divide/1
  Logical Operator/1 -> Sinal_Pulso/1
  Gain/1 -> Relational Operator1/2
  Divide/1 -> Gain1/1, Gain/1, Math Function/2  "Theta_p"
  Constant/1 -> Relational Operator/2
  Relational Operator1/1 -> Logical Operator/2
  Relational Operator/1 -> Logical Operator/1
  Math Function/1 -> Relational Operator/1, Relational Operator1/1
  Add/1 -> Math Function/1
  Theta/1 -> Add/1
  Gain1/1 -> Add/2

== system comparando_simulacoes_rate_diferente_entre_sensor_e_controlador/Controlador discreto (Ts = 0.001) Sensor discreto M (Ts = 0.01)/Encoder/Subsystem ==
  note: Dependendo do sentido da rotaçao, incrementa ou decrementa o contador
  POS : Inport
  NEG : Inport  Port=2
  Constant : Constant  Value=4*Nr
  Conversion : DataTypeConversion  OutDataTypeStr=int32
  Conversion1 : DataTypeConversion  OutDataTypeStr=int32
  Math Function : Math  Operator=mod  SaturateOnIntegerOverflow=on
  Memory : Memory
  Sum : Sum  Inputs=+-+
  Out : Outport
  wires:
  Sum/1 -> Math Function/1
  Memory/1 -> Out/1, Sum/3
  Math Function/1 -> Memory/1
  POS/1 -> Conversion/1
  Conversion/1 -> Sum/1
  Conversion1/1 -> Sum/2
  NEG/1 -> Conversion1/1

== system comparando_simulacoes_rate_diferente_entre_sensor_e_controlador/Controlador discreto (Ts = 0.01) Sensor discreto M (Ts = 0.01)/BLDC1/Cálculo Torque fase "a" ==
  i_a : Inport
  Theta_e : Inport  Port=2
  Constant1 : Constant  Value=360
  Gain : Gain  Gain=Kt/2
  Gain1 : Gain  Gain=180/pi
  Math Function1 : Math  Operator=mod  SaturateOnIntegerOverflow=on
  Product : Product  RndMeth=Zero
  fa1 : Lookup  InputValues=[0 30 60 90 120 150 180 210 240 270 300 330 360]  Table=[ 1 1 1 0 -1 -1 -1 -1 -1 0 1 1 1]
  T_a : Outport
  wires:
  i_a/1 -> Gain/1
  Gain/1 -> Product/2
  Math Function1/1 -> fa1/1
  Theta_e/1 -> Gain1/1
  fa1/1 -> Product/1
  Product/1 -> T_a/1
  Gain1/1 -> Math Function1/1
  Constant1/1 -> Math Function1/2

== system comparando_simulacoes_rate_diferente_entre_sensor_e_controlador/Controlador discreto (Ts = 0.01) Sensor discreto M (Ts = 0.01)/BLDC1/Cálculo Torque fase "b" ==
  i_b : Inport
  Theta_e : Inport  Port=2
  Constant1 : Constant  Value=360
  Gain : Gain  Gain=Kt/2
  Gain1 : Gain  Gain=180/pi
  Math Function1 : Math  Operator=mod  SaturateOnIntegerOverflow=on
  Product : Product  RndMeth=Zero
  fb2 : Lookup  InputValues=[0 30 60 90 120 150 180 210 240 270 300 330 360]  Table=[-1 0 1 1 1 1 1 0 -1 -1 -1 -1 -1]
  T_b : Outport
  wires:
  Product/1 -> T_b/1
  fb2/1 -> Product/1
  Theta_e/1 -> Gain1/1
  Math Function1/1 -> fb2/1
  Gain/1 -> Product/2
  i_b/1 -> Gain/1
  Gain1/1 -> Math Function1/1
  Constant1/1 -> Math Function1/2

== system comparando_simulacoes_rate_diferente_entre_sensor_e_controlador/Controlador discreto (Ts = 0.01) Sensor discreto M (Ts = 0.01)/BLDC1/Cálculo Torque fase "c" ==
  i_c : Inport
  Theta_e : Inport  Port=2
  Constant1 : Constant  Value=360
  Gain : Gain  Gain=Kt/2
  Gain1 : Gain  Gain=180/pi
  Math Function1 : Math  Operator=mod  SaturateOnIntegerOverflow=on
  Product : Product  RndMeth=Zero
  fc1 : Lookup  InputValues=[0 30 60 90 120 150 180 210 240 270 300 330 360]  Table=[-1 -1 -1 -1 -1 0 1 1 1 1 1 0 -1]
  T_c : Outport
  wires:
  i_c/1 -> Gain/1
  Gain/1 -> Product/2
  Math Function1/1 -> fc1/1
  Theta_e/1 -> Gain1/1
  fc1/1 -> Product/1
  Product/1 -> T_c/1
  Gain1/1 -> Math Function1/1
  Constant1/1 -> Math Function1/2

== system comparando_simulacoes_rate_diferente_entre_sensor_e_controlador/Controlador discreto (Ts = 0.01) Sensor discreto M (Ts = 0.01)/BLDC1/Cálculo das FCEMs ==
  Theta_e : Inport
  w_m : Inport  Port=2
  Constant1 : Constant  Value=360
  Constant2 : Constant  Value=360
  Constant3 : Constant  Value=360
  Gain1 : Gain  Gain=180/pi
  Gain2 : Gain  Gain=Ke/2
  Gain3 : Gain  Gain=Ke/2
  Gain4 : Gain  Gain=Ke/2
  Gain5 : Gain  Gain=180/pi
  Gain6 : Gain  Gain=180/pi
  Math Function1 : Math  Operator=mod  SaturateOnIntegerOverflow=on
  Math Function2 : Math  Operator=mod  SaturateOnIntegerOverflow=on
  Math Function3 : Math  Operator=mod  SaturateOnIntegerOverflow=on
  Product : Product  RndMeth=Zero
  Product1 : Product  RndMeth=Zero
  Product2 : Product  RndMeth=Zero
  fa1 : Lookup  InputValues=[0 30 60 90 120 150 180 210 240 270 300 330 360]  Table=[ 1 1 1 0 -1 -1 -1 -1 -1 0 1 1 1]
  fb2 : Lookup  InputValues=[0 30 60 90 120 150 180 210 240 270 300 330 360]  Table=[-1 0 1 1 1 1 1 0 -1 -1 -1 -1 -1]
  fc1 : Lookup  InputValues=[0 30 60 90 120 150 180 210 240 270 300 330 360]  Table=[-1 -1 -1 -1 -1 0 1 1 1 1 1 0 -1]
  e_a : Outport
  e_b : Outport  Port=2
  e_c : Outport  Port=3
  wires:
  fc1/1 -> Gain4/1
  Math Function3/1 -> fc1/1
  fb2/1 -> Gain3/1
  Math Function2/1 -> fb2/1
  fa1/1 -> Gain2/1
  Math Function1/1 -> fa1/1
  Gain6/1 -> Math Function3/1
  Gain5/1 -> Math Function2/1
  Gain1/1 -> Math Function1/1
  Gain4/1 -> Product2/2
  Gain3/1 -> Product1/2
  w_m/1 -> Product2/1, Product1/1, Product/1
  Gain2/1 -> Product/2
  Product2/1 -> e_c/1
  Theta_e/1 -> Gain6/1, Gain1/1, Gain5/1
  Product1/1 -> e_b/1
  Product/1 -> e_a/1
  Constant1/1 -> Math Function1/2
  Constant2/1 -> Math Function2/2
  Constant3/1 -> Math Function3/2

== system comparando_simulacoes_rate_diferente_entre_sensor_e_controlador/Controlador discreto (Ts = 0.01) Sensor discreto M (Ts = 0.01)/BLDC1/Dinâmica fase "a" ==
  note: Gain
  Va : Inport
  e_a : Inport  Port=2
  " " : Gain  Gain=1/L
  Gain : Gain  Gain=R
  Integrator : Integrator
  Sum : Sum  Inputs=+--
  i_a : Outport
  wires:
  Integrator/1 -> i_a/1, Gain/1
  Va/1 -> Sum/1
  Sum/1 -> " "/1
  " "/1 -> Integrator/1
  Gain/1 -> Sum/3
  e_a/1 -> Sum/2

== system comparando_simulacoes_rate_diferente_entre_sensor_e_controlador/Controlador discreto (Ts = 0.01) Sensor discreto M (Ts = 0.01)/BLDC1/Dinâmica fase "b" ==
  note: Gain
  Vb : Inport
  e_b : Inport  Port=2
  " " : Gain  Gain=1/L
  Gain : Gain  Gain=R
  Integrator : Integrator
  Sum : Sum  Inputs=+--
  i_b : Outport
  wires:
  e_b/1 -> Sum/2
  Gain/1 -> Sum/3
  " "/1 -> Integrator/1
  Sum/1 -> " "/1
  Vb/1 -> Sum/1
  Integrator/1 -> Gain/1, i_b/1

== system comparando_simulacoes_rate_diferente_entre_sensor_e_controlador/Controlador discreto (Ts = 0.01) Sensor discreto M (Ts = 0.01)/BLDC1/Dinâmica fase "c" ==
  note: Gain
  Vc : Inport
  e_c : Inport  Port=2
  " " : Gain  Gain=1/L
  Gain : Gain  Gain=R
  Integrator : Integrator
  Sum : Sum  Inputs=+--
  i_c : Outport
  wires:
  Integrator/1 -> i_c/1, Gain/1
  Vc/1 -> Sum/1
  Sum/1 -> " "/1
  " "/1 -> Integrator/1
  Gain/1 -> Sum/3
  e_c/1 -> Sum/2

== system comparando_simulacoes_rate_diferente_entre_sensor_e_controlador/Controlador discreto (Ts = 0.01) Sensor discreto M (Ts = 0.01)/BLDC1/Dinâmica mecânica  ==
  Te : Inport
  Tl : Inport  Port=2
  Gain : Gain  Gain=1/J
  Gain1 : Gain  Gain=Kd
  Integrator : Integrator
  Integrator1 : Integrator
  Sum1 : Sum  Inputs=+--
  Theta_m : Outport
  w_m : Outport  Port=2
  wires:
  Sum1/1 -> Gain/1
  Gain/1 -> Integrator/1
  Integrator/1 -> w_m/1, Integrator1/1, Gain1/1
  Te/1 -> Sum1/1
  Gain1/1 -> Sum1/3
  Tl/1 -> Sum1/2
  Integrator1/1 -> Theta_m/1

== system comparando_simulacoes_rate_diferente_entre_sensor_e_controlador/Controlador discreto (Ts = 0.01) Sensor discreto M (Ts = 0.01)/Encoder/Determinar direçao ==
  note: Dependendo dos valores passados e dos valores atuais
      | dos pulsos de cada sensor óptico, determina o sentido
      | de rotaçao.
  note: 00
      | 01
      | 10
      | 11
  note: 00 01 10 11
  note: 0	-	+	0
      | +	0	0	-
      | -	0	0	+
      | 0	+	-	0
  note: Implementa a seguinte tabela verdade:
  note: AB
  note: A'B'
  note: A,B = Valores atuais dos sinais A e B
      | A'B' = Valores passados do sinais A e B
  A : Inport
  B : Inport  Port=2
  Bus Creator1 : BusCreator
  Combinatorial  Logic : CombinatorialLogic  TruthTable=[ 0 0 ; 0 1 ; 1 0 ; 0 0 ; 1 0 ; 0 0 ; 0 0 ; 0 1 ; 0 1 ; 0 0 ; 0 0 ; 1 0 ; 0 0 ; 1 0 ; 0 1 ; 0 0]
  Demux : Demux  Outputs=2
  Memory : Memory
  Memory1 : Memory
  POS : Outport
  NEG : Outport  Port=2
  wires:
  B/1 -> Bus Creator1/4, Memory1/1
  Memory1/1 -> Bus Creator1/2
  Bus Creator1/1 -> Combinatorial  Logic/1
  Memory/1 -> Bus Creator1/1
  Combinatorial  Logic/1 -> Demux/1
  Demux/2 -> NEG/1
  A/1 -> Bus Creator1/3, Memory/1
  Demux/1 -> POS/1

== system comparando_simulacoes_rate_diferente_entre_sensor_e_controlador/Controlador discreto (Ts = 0.01) Sensor discreto M (Ts = 0.01)/Encoder/Método M ==
  Posição : Inport
  Add : Sum  Inputs=+-|
  Detect Increase : simulink/Logic and Bit Operations/Detect Increase  vinit=0.0  InputProcessing=Inherited  OutDataTypeStr=boolean
  Gain : Gain  Gain=1/Ts
  Memory1 : Memory
  Pulse Generator : DiscretePulseGenerator  PulseType=Time based  Period=Ts  PulseWidth=50
  Switch : Switch
  Switch1 : Switch
  pos' : Memory
  Velocidade : Outport
  wires:
  Detect Increase/1 -> Switch1/2, Switch/2
  Gain/1 -> Switch/1
  Posição/1 -> Add/1, Switch1/1
  Memory1/1 -> Switch/3, Velocidade/1
  Switch/1 -> Memory1/1
  Switch1/1 -> pos'/1
  Add/1 -> Gain/1
  Pulse Generator/1 -> Detect Increase/1
  pos'/1 -> Switch1/3, Add/2

== system comparando_simulacoes_rate_diferente_entre_sensor_e_controlador/Controlador discreto (Ts = 0.01) Sensor discreto M (Ts = 0.01)/Encoder/Método T ==
  A : Inport
  B : Inport  Port=2
  Clock : Clock
  Compare To Constant : simulink/Logic and Bit Operations/Compare To Constant  relop===  const=m  OutDataTypeStr=boolean
  Constant : Constant  Value=m
  Contador : Subsystem
  Detect Change : simulink/Logic and Bit Operations/Detect Change  vinit=0  InputProcessing=Inherited  OutDataTypeStr=boolean
  Detect Change1 : simulink/Logic and Bit Operations/Detect Change  vinit=0  InputProcessing=Inherited  OutDataTypeStr=boolean
  Divide : Product  Inputs=*/
  Gain : Gain  Gain=360/(4*Nr)
  Logical Operator : Logic  Operator=OR  AllPortsSameDT=off  OutDataTypeStr=boolean
  Memória controlavel : Subsystem
  Memória controlavel1 : Subsystem
  Sum : Sum  Inputs=|+-
  Velocidade : Outport
  wires:
  Memória controlavel1/1(Out) -> Velocidade/1
  Compare To Constant/1 -> Memória controlavel/2(ctrl), Contador/2(reset), Memória controlavel1/2(ctrl)
  Clock/1 -> Memória controlavel/1(In), Sum/1
  Gain/1 -> Divide/1
  Sum/1 -> Divide/2
  Memória controlavel/1(Out) -> Sum/2
  Divide/1 -> Memória controlavel1/1(In)
  Constant/1 -> Gain/1
  Contador/1(Count) -> Compare To Constant/1
  Logical Operator/1 -> Contador/1(In)
  Detect Change1/1 -> Logical Operator/2
  Detect Change/1 -> Logical Operator/1
  B/1 -> Detect Change1/1
  A/1 -> Detect Change/1

== system comparando_simulacoes_rate_diferente_entre_sensor_e_controlador/Controlador discreto (Ts = 0.01) Sensor discreto M (Ts = 0.01)/Encoder/Sensor Óptico ==
  note: Saída do sensor óptico é:
      | 1, se	0 < mod(T,Tp) < \frac{Tp}{2}
      |  0, se      Tp/2 < mod(T,Tp) < Tp
  Theta : Inport
  Constant : Constant  Value=0
  Constant1 : Constant  Value=Nr
  Constant2 : Constant  Value=360
  Divide : Product  Inputs=*/
  Gain : Gain  Gain=1/2
  Logical Operator : Logic  AllPortsSameDT=off  OutDataTypeStr=boolean
  Math Function : Math  Operator=mod  SaturateOnIntegerOverflow=on
  Relational Operator : RelationalOperator  Operator=>  OutDataTypeStr=boolean
  Relational Operator1 : RelationalOperator  Operator=<  OutDataTypeStr=boolean
  Sinal_Pulso : Outport
  wires:
  Constant1/1 -> Divide/2
  Constant2/1 -> Divide/1
  Logical Operator/1 -> Sinal_Pulso/1
  Gain/1 -> Relational Operator1/2
  Divide/1 -> Gain/1, Math Function/2  "Theta_p"
  Constant/1 -> Relational Operator/2
  Relational Operator1/1 -> Logical Operator/2
  Relational Operator/1 -> Logical Operator/1
  Theta/1 -> Math Function/1
  Math Function/1 -> Relational Operator/1, Relational Operator1/1

== system comparando_simulacoes_rate_diferente_entre_sensor_e_controlador/Controlador discreto (Ts = 0.01) Sensor discreto M (Ts = 0.01)/Encoder/Sensor Óptico1 ==
  note: Saída do sensor óptico é:
      | 1, se	0 < mod(T-Tp/4,Tp) < Tp/2
      |  0, se     Tp/2 < mod(T-Tp/4,Tp) < Tp
  Theta : Inport
  Add : Sum  Inputs=+-
  Constant : Constant  Value=0
  Constant1 : Constant  Value=Nr
  Constant2 : Constant  Value=360
  Divide : Product  Inputs=*/
  Gain : Gain  Gain=1/2
  Gain1 : Gain  Gain=1/4
  Logical Operator : Logic  AllPortsSameDT=off  OutDataTypeStr=boolean
  Math Function : Math  Operator=mod  SaturateOnIntegerOverflow=on
  Relational Operator : RelationalOperator  Operator=>  OutDataTypeStr=boolean
  Relational Operator1 : RelationalOperator  Operator=<  OutDataTypeStr=boolean
  Sinal_Pulso : Outport
  wires:
  Gain1/1 -> Add/2
  Theta/1 -> Add/1
  Add/1 -> Math Function/1
  Math Function/1 -> Relational Operator1/1, Relational Operator/1
  Relational Operator/1 -> Logical Operator/1
  Relational Operator1/1 -> Logical Operator/2
  Constant/1 -> Relational Operator/2
  Divide/1 -> Math Function/2, Gain/1, Gain1/1  "Theta_p"
  Gain/1 -> Relational Operator1/2
  Logical Operator/1 -> Sinal_Pulso/1
  Constant2/1 -> Divide/1
  Constant1/1 -> Divide/2

== system comparando_simulacoes_rate_diferente_entre_sensor_e_controlador/Controlador discreto (Ts = 0.01) Sensor discreto M (Ts = 0.01)/Encoder/Subsystem ==
  note: Dependendo do sentido da rotaçao, incrementa ou decrementa o contador
  POS : Inport
  NEG : Inport  Port=2
  Constant : Constant  Value=4*Nr
  Conversion : DataTypeConversion  OutDataTypeStr=int32
  Conversion1 : DataTypeConversion  OutDataTypeStr=int32
  Math Function : Math  Operator=mod  SaturateOnIntegerOverflow=on
  Memory : Memory
  Sum : Sum  Inputs=+-+
  Out : Outport
  wires:
  NEG/1 -> Conversion1/1
  Conversion1/1 -> Sum/2
  Conversion/1 -> Sum/1
  POS/1 -> Conversion/1
  Math Function/1 -> Memory/1
  Memory/1 -> Sum/3, Out/1
  Sum/1 -> Math Function/1

== system comparando_simulacoes_rate_diferente_entre_sensor_e_controlador/Controle contínuo Sensor instantâneo/BLDC/Cálculo Torque fase "a" ==
  i_a : Inport
  Theta_e : Inport  Port=2
  Constant1 : Constant  Value=360
  Gain : Gain  Gain=Kt/2
  Gain1 : Gain  Gain=180/pi
  Math Function1 : Math  Operator=mod  SaturateOnIntegerOverflow=on
  Product : Product  RndMeth=Zero
  fa1 : Lookup  InputValues=[0 30 60 90 120 150 180 210 240 270 300 330 360]  Table=[ 1 1 1 0 -1 -1 -1 -1 -1 0 1 1 1]
  T_a : Outport
  wires:
  i_a/1 -> Gain/1
  Gain/1 -> Product/2
  Math Function1/1 -> fa1/1
  Theta_e/1 -> Gain1/1
  fa1/1 -> Product/1
  Product/1 -> T_a/1
  Gain1/1 -> Math Function1/1
  Constant1/1 -> Math Function1/2

== system comparando_simulacoes_rate_diferente_entre_sensor_e_controlador/Controle contínuo Sensor instantâneo/BLDC/Cálculo Torque fase "b" ==
  i_b : Inport
  Theta_e : Inport  Port=2
  Constant1 : Constant  Value=360
  Gain : Gain  Gain=Kt/2
  Gain1 : Gain  Gain=180/pi
  Math Function1 : Math  Operator=mod  SaturateOnIntegerOverflow=on
  Product : Product  RndMeth=Zero
  fb2 : Lookup  InputValues=[0 30 60 90 120 150 180 210 240 270 300 330 360]  Table=[-1 0 1 1 1 1 1 0 -1 -1 -1 -1 -1]
  T_b : Outport
  wires:
  Product/1 -> T_b/1
  fb2/1 -> Product/1
  Theta_e/1 -> Gain1/1
  Math Function1/1 -> fb2/1
  Gain/1 -> Product/2
  i_b/1 -> Gain/1
  Gain1/1 -> Math Function1/1
  Constant1/1 -> Math Function1/2

== system comparando_simulacoes_rate_diferente_entre_sensor_e_controlador/Controle contínuo Sensor instantâneo/BLDC/Cálculo Torque fase "c" ==
  i_c : Inport
  Theta_e : Inport  Port=2
  Constant1 : Constant  Value=360
  Gain : Gain  Gain=Kt/2
  Gain1 : Gain  Gain=180/pi
  Math Function1 : Math  Operator=mod  SaturateOnIntegerOverflow=on
  Product : Product  RndMeth=Zero
  fc1 : Lookup  InputValues=[0 30 60 90 120 150 180 210 240 270 300 330 360]  Table=[-1 -1 -1 -1 -1 0 1 1 1 1 1 0 -1]
  T_c : Outport
  wires:
  i_c/1 -> Gain/1
  Gain/1 -> Product/2
  Math Function1/1 -> fc1/1
  Theta_e/1 -> Gain1/1
  fc1/1 -> Product/1
  Product/1 -> T_c/1
  Gain1/1 -> Math Function1/1
  Constant1/1 -> Math Function1/2

== system comparando_simulacoes_rate_diferente_entre_sensor_e_controlador/Controle contínuo Sensor instantâneo/BLDC/Cálculo das FCEMs ==
  Theta_e : Inport
  w_m : Inport  Port=2
  Constant1 : Constant  Value=360
  Constant2 : Constant  Value=360
  Constant3 : Constant  Value=360
  Gain1 : Gain  Gain=180/pi
  Gain2 : Gain  Gain=Ke/2
  Gain3 : Gain  Gain=Ke/2
  Gain4 : Gain  Gain=Ke/2
  Gain5 : Gain  Gain=180/pi
  Gain6 : Gain  Gain=180/pi
  Math Function1 : Math  Operator=mod  SaturateOnIntegerOverflow=on
  Math Function2 : Math  Operator=mod  SaturateOnIntegerOverflow=on
  Math Function3 : Math  Operator=mod  SaturateOnIntegerOverflow=on
  Product : Product  RndMeth=Zero
  Product1 : Product  RndMeth=Zero
  Product2 : Product  RndMeth=Zero
  fa1 : Lookup  InputValues=[0 30 60 90 120 150 180 210 240 270 300 330 360]  Table=[ 1 1 1 0 -1 -1 -1 -1 -1 0 1 1 1]
  fb2 : Lookup  InputValues=[0 30 60 90 120 150 180 210 240 270 300 330 360]  Table=[-1 0 1 1 1 1 1 0 -1 -1 -1 -1 -1]
  fc1 : Lookup  InputValues=[0 30 60 90 120 150 180 210 240 270 300 330 360]  Table=[-1 -1 -1 -1 -1 0 1 1 1 1 1 0 -1]
  e_a : Outport
  e_b : Outport  Port=2
  e_c : Outport  Port=3
  wires:
  fc1/1 -> Gain4/1
  Math Function3/1 -> fc1/1
  fb2/1 -> Gain3/1
  Math Function2/1 -> fb2/1
  fa1/1 -> Gain2/1
  Math Function1/1 -> fa1/1
  Gain6/1 -> Math Function3/1
  Gain5/1 -> Math Function2/1
  Gain1/1 -> Math Function1/1
  Gain4/1 -> Product2/2
  Gain3/1 -> Product1/2
  w_m/1 -> Product2/1, Product1/1, Product/1
  Gain2/1 -> Product/2
  Product2/1 -> e_c/1
  Theta_e/1 -> Gain6/1, Gain1/1, Gain5/1
  Product1/1 -> e_b/1
  Product/1 -> e_a/1
  Constant1/1 -> Math Function1/2
  Constant2/1 -> Math Function2/2
  Constant3/1 -> Math Function3/2

== system comparando_simulacoes_rate_diferente_entre_sensor_e_controlador/Controle contínuo Sensor instantâneo/BLDC/Dinâmica fase "a" ==
  note: Gain
  Va : Inport
  e_a : Inport  Port=2
  " " : Gain  Gain=1/L
  Gain : Gain  Gain=R
  Integrator : Integrator
  Sum : Sum  Inputs=+--
  i_a : Outport
  wires:
  Integrator/1 -> i_a/1, Gain/1
  Va/1 -> Sum/1
  Sum/1 -> " "/1
  " "/1 -> Integrator/1
  Gain/1 -> Sum/3
  e_a/1 -> Sum/2

== system comparando_simulacoes_rate_diferente_entre_sensor_e_controlador/Controle contínuo Sensor instantâneo/BLDC/Dinâmica fase "b" ==
  note: Gain
  Vb : Inport
  e_b : Inport  Port=2
  " " : Gain  Gain=1/L
  Gain : Gain  Gain=R
  Integrator : Integrator
  Sum : Sum  Inputs=+--
  i_b : Outport
  wires:
  e_b/1 -> Sum/2
  Gain/1 -> Sum/3
  " "/1 -> Integrator/1
  Sum/1 -> " "/1
  Vb/1 -> Sum/1
  Integrator/1 -> Gain/1, i_b/1
